simulink model "TRAMI_STEP_AT_vehicle_ver01_Jmaab_R2018b_Intg"  (R2018b)
settings: Solver=ode8  StartTime=0  StopTime=end_time  FixedStep=sampling_time  RelTol=1e-3
PreLoadFcn:
  | %init_setting;
values from neighbouring files (symbols this model uses):
  sampling_time = 0.0025    [METI_TRAMI_Thermal_ver01_Jmaab_PreLoad.m]
undefined symbols (not defined in the file or in its folder): ACC_D_Gain, ACC_I_Gain, ACC_P_Gain, ALT_CNT_ALT_OFF_RPM_HYS_rpm, ALT_CNT_ALT_ON_RPM_HYS_rpm, ALT_CNT_Alter_V_BASE_V, ALT_CNT_Alter_V_Kaisei_V, ALT_CNT_flag_disable_kaisei, ALT_CNT_V_Battely_Kudo_V, ALT_PNT_ALT_GDCurrent_A, ALT_PNT_ALT_GDVolt_V, ALT_PNT_Alter_limit_Current_V_table, ALT_PNT_Alter_limit_Current_V_table_x_rpm, ALT_PNT_Alter_trq_Nm_map, ALT_PNT_Alter_trq_Nm_map_x_rpm, ALT_PNT_Alter_trq_Nm_map_y_Current_A, ALT_PNT_Alter_trq_Nm_map_z_Volt_tgt_V, ALT_PNT_eta_pulley_alt, ALT_PNT_Gain_Alt_v_del, ALT_PNT_ratio_pulley_alt, ALT_PNT_Tau_Alternator_V_tgt_s, ALT_PNT_trq_alter_output_LL_Nm, BK_PNT_Pow_UL, BK_PNT_Tau_brake, Brk_LL, Brk_PGain, Brk_UL, BT_PNT_Lo_Capa_lo_batt_F, BT_PNT_Lo_ocv_SOC_lo_batt_OCV_V_table, BT_PNT_Lo_ocv_SOC_lo_batt_OCV_V_table_x_SOC, BT_PNT_Lo_R_lo_batt_ohm, BT_PNT_Lo_SOC_MAX_lo_batt, BT_PNT_Lo_SOC_MIN_lo_batt, BT_PNT_Lo_SOC_START_lo_batt, BT_PNT_Lo_V_start_ocv, Driver_Brake_Const1, Driver_Brake_Const3, Driver_Brake_Switch_Const2, Driver_Brk_sh, drivmode_ACC, drivmode_CONST, drivmode_GensokuKaisei, drivmode_GensokuRikko, drivmode_STOP, EL_PNT_R_bodyelec_lo_ohm, ENG_CNT_Accel_LL, ENG_CNT_Accel_UL, ENG_CNT_brak_idlestop, ENG_CNT_flag_idle_stop_exe, ENG_CNT_gain_p_per_isc, ENG_CNT_IdleSpeed_Const, ENG_CNT_omg_eng_fuelcut_rpm, ENG_CNT_per_isc_max, ENG_CNT_per_isc_min, ENG_CNT_per_throttle_fuelcut, ENG_CNT_per_throttle_isc_fb, ENG_CNT_Starter_timer_Const_s, ENG_CNT_Throttle_LL, ENG_CNT_Throttle_UL, ENG_CNT_V_car_idlestop_kmph ... (+29)
libraries: METI_Lib_vehicle_model x18, simulink x4, AZAPA_Lib_vehicle_model x1
(part 1 of 3)
settings Model: SimulationMode=accelerator  Creator=nishimura  LastModifiedBy=E00026
settings DataIOCC: LimitDataPoints=on  SaveFormat=Array  InspectSignalLogs=on
settings OptimizationCC: BlockReduction=off  BooleanDataType=off  LifeSpan=inf
settings DebuggingCC: SaveWithParameterizedLinksMsg=none  UnderspecifiedInitializationDetection=Classic  MergeDetectMultiDrivingBlocksExec=none  SignalResolutionControl=TryResolveAllWithWarning  ParameterPrecisionLossMsg=none  StrictBusMsg=ErrorOnBusTreatedAsVector  SFUnexpectedBacktrackingDiag=warning  SFNoUnconditionalDefaultTransitionDiag=warning  SFExecutionAtInitializationDiag=none
settings HardwareCC: ProdBitPerPointer=32  ProdBitPerSizeT=32  ProdBitPerPtrDiffT=32  ProdLargestAtomicFloat=None  ProdIntDivRoundTo=Undefined  ProdEndianess=Unspecified  ProdWordSize=32  ProdHWDeviceType=32-bit Generic  TargetUnknown=on
settings ModelReferenceCC: PropagateSignalLabelsOutOfModel=off
settings SFSimCC: SimUseLocalCustomCode=off
settings RTWCC: RTWUseLocalCustomCode=off
settings CodeAppCC: StateflowObjectComments=on
settings GRTTargetCC: TargetLangStandard=C89/C90 (ANSI)  GeneratePreprocessorConditionals=Disable all
settings ConfigComp: CovMetricSettings=dw  CovHtmlReporting=on  CovSaveCumulativeToWorkspaceVar=on  CovSaveSingleToWorkspaceVar=on  CovExternalEMLEnable=off  CovSFcnEnable=off

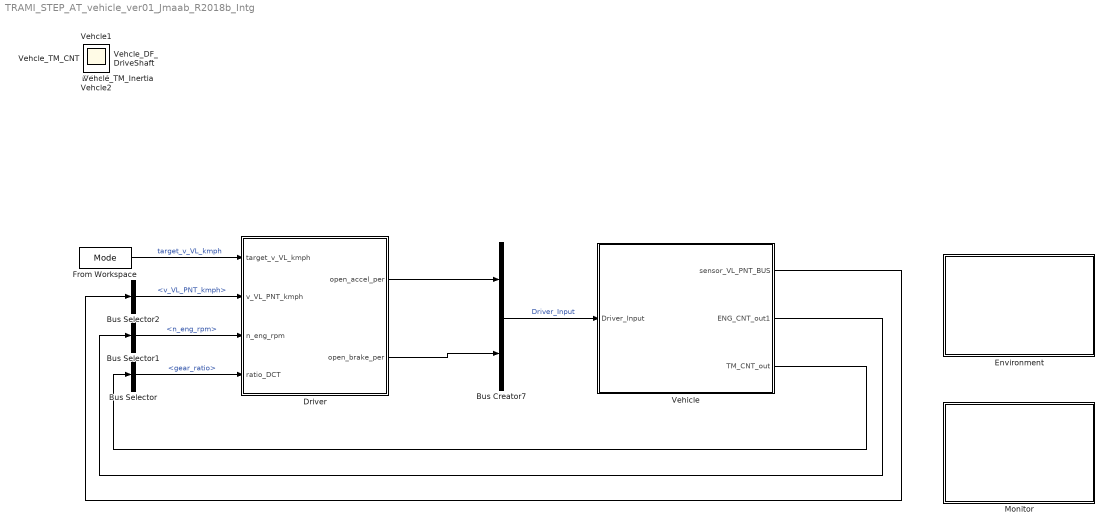
== system TRAMI_STEP_AT_vehicle_ver01_Jmaab_R2018b_Intg ==
  Bus Creator7 : BusCreator  Inputs=2
  Bus Selector : BusSelector  OutputSignals=gear_ratio
  Bus Selector1 : BusSelector  OutputSignals=n_eng_rpm
  Bus Selector2 : BusSelector  OutputSignals=v_VL_PNT_kmph
  Driver : Subsystem
      mask Display: image(imread('picture\driver.png'))
  Environment : Subsystem
      mask Display: image(imread('picture\environment.png'))
  From Workspace : FromWorkspace  VariableName=Mode  SampleTime=0  OutputAfterFinalValue=Holding final value
  Monitor : Subsystem
  Vehicle : Subsystem
      mask Display: image(imread('picture\electric_load.png'))
  Driver1 : Scope
  Vehcle1 : Scope
  Vehcle2 : Scope
  Vehcle_DF_DriveShaft : Scope
  Vehcle_TM_CNT : Scope
  Vehcle_TM_Inertia : Scope
  wires:
  From Workspace/1 -> Driver/1(target_v_VL_kmph)  "target_v_VL_kmph"
  Bus Creator7/1 -> Vehicle/1(Driver_Input)  "Driver_Input"
  Vehicle/1(sensor_VL_PNT_BUS) -> Bus Selector2/1
  Vehicle/3(TM_CNT_out) -> Bus Selector/1
  Vehicle/2(ENG_CNT_out1) -> Bus Selector1/1
  Driver/1(open_accel_per) -> Bus Creator7/1
  Driver/2(open_brake_per) -> Bus Creator7/2
  Bus Selector/1 -> Driver/4(ratio_DCT)  "<gear_ratio>"
  Bus Selector1/1 -> Driver/3(n_eng_rpm)  "<n_eng_rpm>"
  Bus Selector2/1 -> Driver/2(v_VL_PNT_kmph)  "<v_VL_PNT_kmph>"

== system TRAMI_STEP_AT_vehicle_ver01_Jmaab_R2018b_Intg/Driver ==
  note: ドライバモデルのへたくそ対応
  note: 全体としてパワーを算出しておいて、
      | さらにパワーと速度のF/Bを切り替えれるようにしておく
  target_v_VL_kmph : Inport
  v_VL_PNT_kmph : Inport  Port=2
  n_eng_rpm : Inport  Port=3
  ratio_DCT : Inport  Port=4
  Caliculate_Driving_State : Subsystem
  Caliculate_Opeining_Accel : Subsystem
  Caliculate_Opening_Brake : Subsystem
  Memory2 : Memory  InheritSampleTime=on
  Memory3 : Memory
  Memory4 : Memory
  open_accel_per : Outport
  open_brake_per : Outport  Port=2
  tag scope: tScope_accel=global, tScope_brake=global
  wires:
  target_v_VL_kmph/1 -> Caliculate_Opeining_Accel/2(target_v_VL_kmph), Caliculate_Opening_Brake/2(target_v_VL_kmph), Caliculate_Driving_State/2(target_v_VL_kmph)
  Memory3/1 -> Caliculate_Opeining_Accel/3(pre_n_eng_rpm)  "pre_n_eng_rpm"
  Memory4/1 -> Caliculate_Opeining_Accel/4(pre_ratio_DCT)
  n_eng_rpm/1 -> Memory3/1
  Memory2/1 -> Caliculate_Opening_Brake/1(v_VL_PNT_kmph), Caliculate_Opeining_Accel/1(v_VL_PNT_kmph)
  Caliculate_Opening_Brake/1(open_brake_per) -> open_brake_per/1, [tScope_brake], Caliculate_Driving_State/1(open_brake_per)
  v_VL_PNT_kmph/1 -> Memory2/1
  ratio_DCT/1 -> Memory4/1
  Caliculate_Opeining_Accel/1(open_accel_per) -> [tScope_accel], open_accel_per/1, Caliculate_Opening_Brake/3(open_accel_per)

== system TRAMI_STEP_AT_vehicle_ver01_Jmaab_R2018b_Intg/Environment ==
  note: 登坂。風、温度、湿度・・・
  Clock : Clock
  To Workspace : ToWorkspace  VariableName=simtime  SampleTime=-1
      settings: Decimation=num_tws_mabiki
  wires:
  Clock/1 -> To Workspace/1

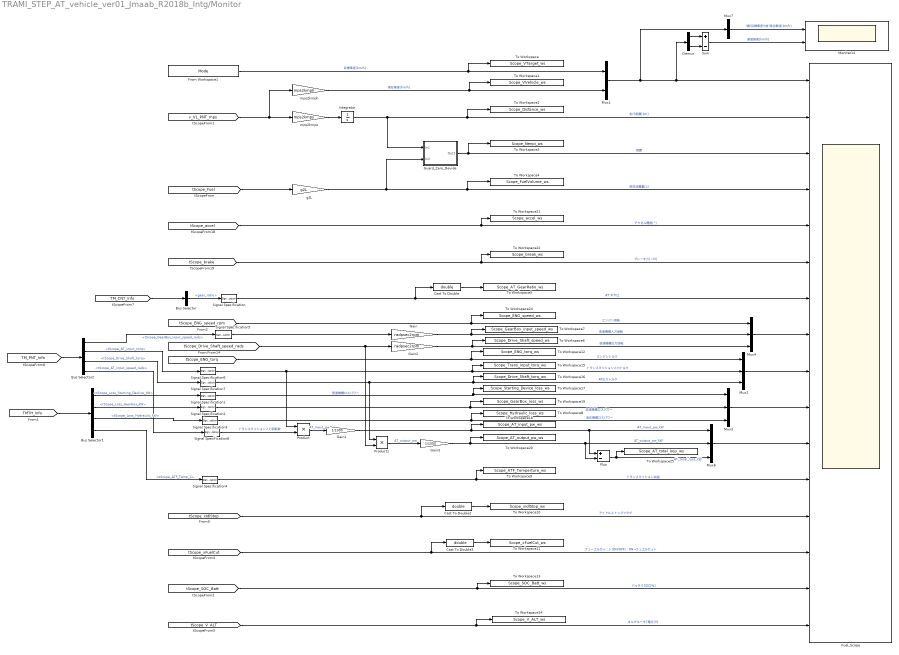
== system TRAMI_STEP_AT_vehicle_ver01_Jmaab_R2018b_Intg/Monitor ==
  Bus Selector : BusSelector  OutputSignals=gear_ratio
  Bus Selector1 : BusSelector  OutputSignals=tScope_Loss_Starting_Deviice_kW,tScope_Loss_Gearbox_kW,tScope_Loss_Hydraulic_kW,tScope_ATF_Temp_C
  Bus Selector2 : BusSelector  OutputSignals=tScope_GearBox_input_speed_rads,tScope_AT_input_torq,tScope_Drive_Shaft_torq,tScope_AT_input_speed_rads
  Cast To Double : DataTypeConversion  OutDataTypeStr=double
  Cast To Double2 : DataTypeConversion  OutDataTypeStr=double
  Cast To Double3 : DataTypeConversion  OutDataTypeStr=double
  Demux : Demux  Outputs=2
  From Workspace1 : FromWorkspace  VariableName=Mode  SampleTime=0  OutputAfterFinalValue=Holding final value
  Fuel_Scope : Scope  NumInputPorts=16
  Gain : Gain  Tag=単位変換  Gain=radpsec2rpm
  Gain1 : Gain  Gain=1/1000
  Gain2 : Gain  Tag=単位変換  Gain=radpsec2rpm
  Gain3 : Gain  Gain=1/1000
  Guard_Zero_Devide : Subsystem
  Integrator : Integrator
  Moniter14 : Scope  NumInputPorts=2
  Mux1 : Mux  Inputs=2
  Mux{2..4,6} (4 alike) : Mux  Inputs=3
  Mux7 : Mux  Inputs=1
  Plus : Sum  Inputs=+-
  Product : Product
  Product1 : Product
  Signal Specification{,1..8} (9 alike) : SignalSpecification
  Sum : Sum  Inputs=+-
  To Workspace : ToWorkspace  VariableName=Scope_VTarget_ws  SampleTime=-1
      settings: Decimation=num_tws_mabiki
  To Workspace1 : ToWorkspace  VariableName=Scope_VVehicle_ws  SampleTime=-1
      settings: Decimation=num_tws_mabiki
  To Workspace10 : ToWorkspace  VariableName=Scope_xIdlStop_ws  SampleTime=-1
      settings: Decimation=num_tws_mabiki
  To Workspace11 : ToWorkspace  VariableName=Scope_xFuelCut_ws  SampleTime=-1
      settings: Decimation=num_tws_mabiki
  To Workspace12 : ToWorkspace  VariableName=Scope_ENG_torq_ws  SampleTime=-1
      settings: Decimation=num_tws_mabiki
  To Workspace13 : ToWorkspace  VariableName=Scope_SOC_Batt_ws  SampleTime=-1
      settings: Decimation=num_tws_mabiki
  To Workspace14 : ToWorkspace  VariableName=Scope_V_ALT_ws  SampleTime=-1
      settings: Decimation=num_tws_mabiki
  To Workspace15 : ToWorkspace  VariableName=Scope_Trans_input_torq_ws  SampleTime=-1
      settings: Decimation=num_tws_mabiki
  To Workspace16 : ToWorkspace  VariableName=Scope_Drive_Shaft_torq_ws  SampleTime=-1
      settings: Decimation=num_tws_mabiki
  To Workspace17 : ToWorkspace  VariableName=Scope_Starting_Device_loss_ws  SampleTime=-1
      settings: Decimation=num_tws_mabiki
  To Workspace18 : ToWorkspace  VariableName=Scope_AT_input_pw_ws  SampleTime=-1
      settings: Decimation=num_tws_mabiki
  To Workspace19 : ToWorkspace  VariableName=Scope_GearBox_loss_ws  SampleTime=-1
      settings: Decimation=num_tws_mabiki
  To Workspace2 : ToWorkspace  VariableName=Scope_Distance_ws  SampleTime=-1
      settings: Decimation=num_tws_mabiki
  To Workspace20 : ToWorkspace  VariableName=Scope_AT_output_pw_ws  SampleTime=-1
      settings: Decimation=num_tws_mabiki
  To Workspace21 : ToWorkspace  VariableName=Scope_accel_ws  SampleTime=-1
      settings: Decimation=num_tws_mabiki
  To Workspace22 : ToWorkspace  VariableName=Scope_break_ws  SampleTime=-1
      settings: Decimation=num_tws_mabiki
  To Workspace24 : ToWorkspace  VariableName=Scope_ENG_speed_ws  SampleTime=-1
      settings: Decimation=num_tws_mabiki
  To Workspace25 : ToWorkspace  VariableName=Scope_AT_total_loss_ws  SampleTime=-1
      settings: Decimation=num_tws_mabiki
  To Workspace3 : ToWorkspace  VariableName=Scope_Nenpi_ws  SampleTime=-1
      settings: Decimation=num_tws_mabiki
  To Workspace4 : ToWorkspace  VariableName=Scope_FuelVolume_ws  SampleTime=-1
      settings: Decimation=num_tws_mabiki
  To Workspace5 : ToWorkspace  VariableName=Scope_AT_GearRatio_ws  SampleTime=-1
      settings: Decimation=num_tws_mabiki
  To Workspace6 : ToWorkspace  VariableName=Scope_Drive_Shaft_speed_ws  SampleTime=-1
      settings: Decimation=num_tws_mabiki
  To Workspace7 : ToWorkspace  VariableName=Scope_GearBox_input_speed_ws  SampleTime=-1
      settings: Decimation=num_tws_mabiki
  To Workspace8 : ToWorkspace  VariableName=Scope_Hydraulic_loss_ws  SampleTime=-1
      settings: Decimation=num_tws_mabiki
  To Workspace9 : ToWorkspace  VariableName=Scope_ATF_Temperture_ws  SampleTime=-1
      settings: Decimation=num_tws_mabiki
  g2L : Gain  Gain=g2L
  mps2kmph : Gain  Gain=mps2kmph
  mps2kmps : Gain  Gain=mps2kmps
  wires:
  [tScope_xFuelCut] -> Fuel_Scope/14, Cast To Double3/1  "フューエルカット[ON/OFF] : ON→フュエルカット"
  [v_VL_PNT_mps] -> mps2kmph/1, mps2kmps/1
  mps2kmps/1 -> Integrator/1
  [tScope_Fuel] -> g2L/1
  Integrator/1 -> Guard_Zero_Devide/1(In1), Fuel_Scope/2, To Workspace2/1  "走行距離[km]"
  g2L/1 -> Fuel_Scope/4, To Workspace4/1, Guard_Zero_Devide/2(In2)  "燃料消費量[L]"
  Signal Specification4/1 -> Fuel_Scope/12, To Workspace9/1  "トランスミッション油温"
  From Workspace1/1 -> To Workspace/1, Mux1/1  "目標車速[km/h]"
  mps2kmph/1 -> To Workspace1/1, Mux1/2  "現在車速[km/h]"
  Mux1/1 -> Mux7/1, Fuel_Scope/1, Demux/1
  Signal Specification2/1 -> To Workspace19/1, Mux3/2  "変速機構ロスパワー"
  Signal Specification7/1 -> Product1/1, To Workspace16/1, Mux2/3  "AT出力トルク"
  Mux3/1 -> Fuel_Scope/10
  [tScope_accel] -> Fuel_Scope/5, To Workspace21/1  "アクセル開度[°]"
  [tScope_brake] -> Fuel_Scope/6, To Workspace22/1  "ブレーキ力[１N]"
  [tScope_ENG_speed_rpm] -> To Workspace24/1, Mux4/1  "エンジン回転"
  Demux/1 -> Sum/1
  Demux/2 -> Sum/2
  Sum/1 -> Moniter14/2  "速度誤差[km/h]"
  [tScope_V_ALT] -> Fuel_Scope/16, To Workspace14/1  "オルタネータ7電圧[V]"
  [tScope_SOC_Batt] -> Fuel_Scope/15, To Workspace13/1  "バッテリSOC[%]"
  Guard_Zero_Devide/1(Out1) -> Fuel_Scope/3, To Workspace3/1  "燃費"
  Gain/1 -> Mux4/2, To Workspace7/1  "変速機構入力回転"
  [tScope_ENG_torq] -> To Workspace12/1, Mux2/1  "エンジントルク"
  Signal Specification6/1 -> Mux2/2, To Workspace15/1, Product/1  "トランスミッション入力トルク"
  Signal Specification1/1 -> To Workspace17/1, Mux3/1  "発進機構ロスパワー"
  Signal Specification3/1 -> To Workspace8/1, Mux3/3  "油圧機構ロスパワー"
  Mux2/1 -> Fuel_Scope/9
  [tScope_xIdlStop] -> Fuel_Scope/13, Cast To Double2/1  "アイドルストップフラグ"
  Mux4/1 -> Fuel_Scope/8
  Cast To Double3/1 -> To Workspace11/1
  Cast To Double2/1 -> To Workspace10/1
  Signal Specification5/1 -> Gain/1
  Gain2/1 -> To Workspace6/1, Mux4/3  "変速機構出力回転"
  [tScope_Drive_Shaft_speed_rads] -> Product1/2, Gain2/1
  Mux6/1 -> Fuel_Scope/11
  Gain1/1 -> To Workspace18/1, Mux6/1, Plus/1  "AT_Input_pw_kW"
  Signal Specification8/1 -> Product/2  "トランスミッション入力回転数"
  Product1/1 -> Gain3/1  "AT_output_pw"
  Plus/1 -> To Workspace25/1, Mux6/3  "AT_total_loss_kW"
  Product/1 -> Gain1/1  "AT_Input_pw"
  Gain3/1 -> To Workspace20/1, Plus/2, Mux6/2  "AT_output_pw_kW"
  Cast To Double/1 -> To Workspace5/1
  Signal Specification/1 -> Cast To Double/1, Fuel_Scope/7  "AT ギヤ比"
  Mux7/1 -> Moniter14/1  "(黄)目標車速/(桃)現在車速[km/h]"
  [TM_CNT_Info] -> Bus Selector/1
  Bus Selector/1 -> Signal Specification/1  "<gear_ratio>"
  [TMTH_Info] -> Bus Selector1/1
  Bus Selector1/1 -> Signal Specification1/1  "<tScope_Loss_Starting_Deviice_kW>"
  Bus Selector1/2 -> Signal Specification2/1  "<tScope_Loss_Gearbox_kW>"
  Bus Selector1/3 -> Signal Specification3/1  "<tScope_Loss_Hydraulic_kW>"
  Bus Selector1/4 -> Signal Specification4/1  "<tScope_ATF_Temp_C>"
  [TM_PNT_Info] -> Bus Selector2/1
  Bus Selector2/1 -> Signal Specification5/1  "<tScope_GearBox_input_speed_rads>"
  Bus Selector2/2 -> Signal Specification6/1  "<tScope_AT_input_torq>"
  Bus Selector2/3 -> Signal Specification7/1  "<tScope_Drive_Shaft_torq>"
  Bus Selector2/4 -> Signal Specification8/1  "<tScope_AT_input_speed_rads>"

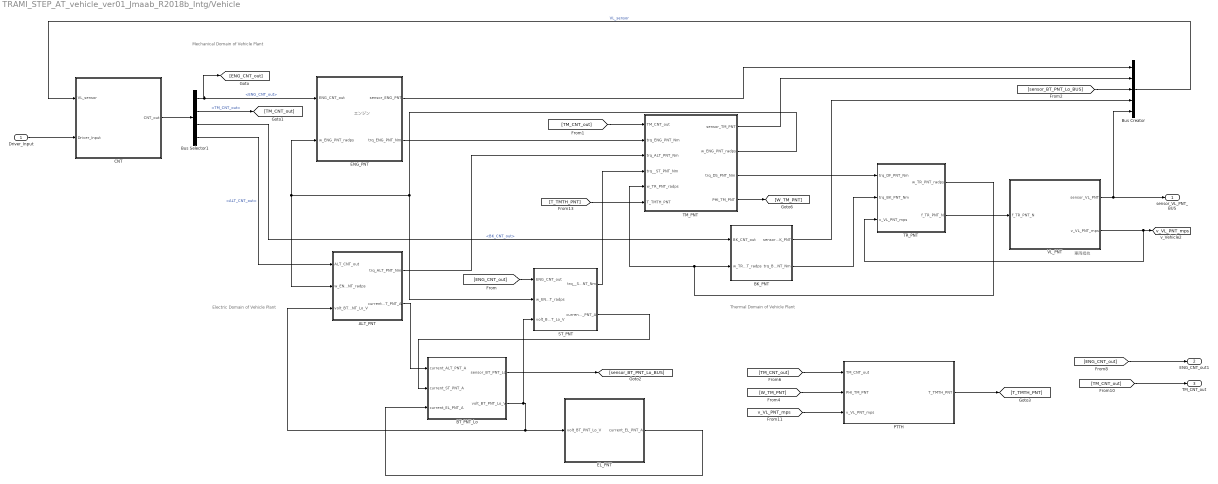
== system TRAMI_STEP_AT_vehicle_ver01_Jmaab_R2018b_Intg/Vehicle ==
  note: エンジン
  note: 車両抵抗
  note: Mechanical Domain of Vehicle Plant
  note: Electric Domain
      |  of Vehicle Plant
  note: Thermal Domain of Vehicle Plant
  Driver_Input : Inport
  ALT_PNT : Subsystem
      mask Display: image(imread('picture\image\alternator02.jpg'))
  BK_PNT : Subsystem
      mask Display: image(imread('picture\brake02.png'))
  BT_PNT_Lo : Subsystem
      mask Display: image(imread('picture\battery.png'))
  Bus Creator : BusCreator  Inputs=5
  Bus Selector1 : BusSelector  OutputSignals=ENG_CNT_out,TM_CNT_out,BK_CNT_out,ALT_CNT_out
  CNT : Subsystem
      mask Display: image(imread('picture\ECU.png'))
  EL_PNT : Subsystem
      mask Display: image(imread('picture\electric_load.png'))
  ENG_PNT : Subsystem
      mask Display: image(imread('picture\image\engine03.jpg'))
  PTTH : Subsystem
  ST_PNT : Subsystem
      mask Display: image(imread('picture\image\starter02.jpg'))
  TM_PNT : Subsystem
  TR_PNT : Subsystem
      mask Display: image(imread('picture\tyre01.png'))
  VL_PNT : Subsystem
      mask Display: image(imread('picture\vehicle_resistance.png'))
  sensor_VL_PNT_BUS : Outport
  ENG_CNT_out1 : Outport  Port=2
  TM_CNT_out : Outport  Port=3
  tag scope: v_VL_PNT_mps=global
  wires:
  ENG_PNT/1(sensor_ENG_PNT) -> Bus Creator/1
  ALT_PNT/1(trq_ALT_PNT_Nm) -> TM_PNT/3(trq_ALT_PNT_Nm)
  EL_PNT/1(current_EL_PNT_A) -> BT_PNT_Lo/3(current_EL_PNT_A)
  ALT_PNT/2(current_ALT_PNT_A) -> BT_PNT_Lo/1(current_ALT_PNT_A)
  ST_PNT/2(current_ST_PNT_A) -> BT_PNT_Lo/2(current_ST_PNT_A)
  BT_PNT_Lo/2(volt_BT_PNT_Lo_V) -> ST_PNT/3(volt_BT_PNT_Lo_V), ALT_PNT/3(volt_BT_PNT_Lo_V), EL_PNT/1(volt_BT_PNT_Lo_V)
  TM_PNT/1(sensor_TM_PNT) -> Bus Creator/2
  ENG_PNT/2(trq_ENG_PNT_Nm) -> TM_PNT/2(trq_ENG_PNT_Nm)
  TM_PNT/2(w_ENG_PNT_radps) -> ALT_PNT/2(w_ENG_PNT_radps), ENG_PNT/2(w_ENG_PNT_radps), ST_PNT/2(w_ENG_PNT_radps)
  ST_PNT/1(trq__ST_PNT_Nm) -> TM_PNT/4(trq__ST_PNT_Nm)
  VL_PNT/1(sensor_VL_PNT) -> sensor_VL_PNT_BUS/1, Bus Creator/5
  TM_PNT/3(trq_DS_PNT_Nm) -> TR_PNT/1(trq_DF_PNT_Nm)
  BK_PNT/2(trq_BK_PNT_Nm) -> TR_PNT/2(trq_BK_PNT_Nm)
  TR_PNT/2(f_TR_PNT_N) -> VL_PNT/1(f_TR_PNT_N)
  TR_PNT/1(w_TR_PNT_radps) -> TM_PNT/5(w_TR_PNT_radps), BK_PNT/2(w_TR_PNT_radps)
  VL_PNT/2(v_VL_PNT_mps) -> TR_PNT/3(v_VL_PNT_mps), [v_VL_PNT_mps]
  [TM_CNT_out] -> TM_CNT_out/1
  Bus Selector1/1 -> [ENG_CNT_out], ENG_PNT/1(ENG_CNT_out)  "<ENG_CNT_out>"
  Bus Selector1/4 -> ALT_PNT/1(ALT_CNT_out)  "<ALT_CNT_out>"
  Bus Selector1/3 -> BK_PNT/1(BK_CNT_out)  "<BK_CNT_out>"
  Bus Creator/1 -> CNT/1(VL_sensor)  "VL_sensor"
  CNT/1(CNT_out) -> Bus Selector1/1
  [ENG_CNT_out] -> ST_PNT/1(ENG_CNT_out)
  Bus Selector1/2 -> [TM_CNT_out]  "<TM_CNT_out>"
  [TM_CNT_out] -> TM_PNT/1(TM_CNT_out)
  BT_PNT_Lo/1(sensor_BT_PNT_Lo) -> [sensor_BT_PNT_Lo_BUS]
  [sensor_BT_PNT_Lo_BUS] -> Bus Creator/3
  Driver_Input/1 -> CNT/2(Driver_Input)
  [ENG_CNT_out] -> ENG_CNT_out1/1
  PTTH/1(T_TMTH_PNT) -> [T_TMTH_PNT]
  [TM_CNT_out] -> PTTH/1(TM_CNT_out)
  [W_TM_PNT] -> PTTH/2(PHI_TM_PNT)
  [v_VL_PNT_mps] -> PTTH/3(v_VL_PNT_mps)
  TM_PNT/4(PHI_TM_PNT) -> [W_TM_PNT]
  [T_TMTH_PNT] -> TM_PNT/6(T_TMTH_PNT)
  BK_PNT/1(sensor_BK_PNT) -> Bus Creator/4

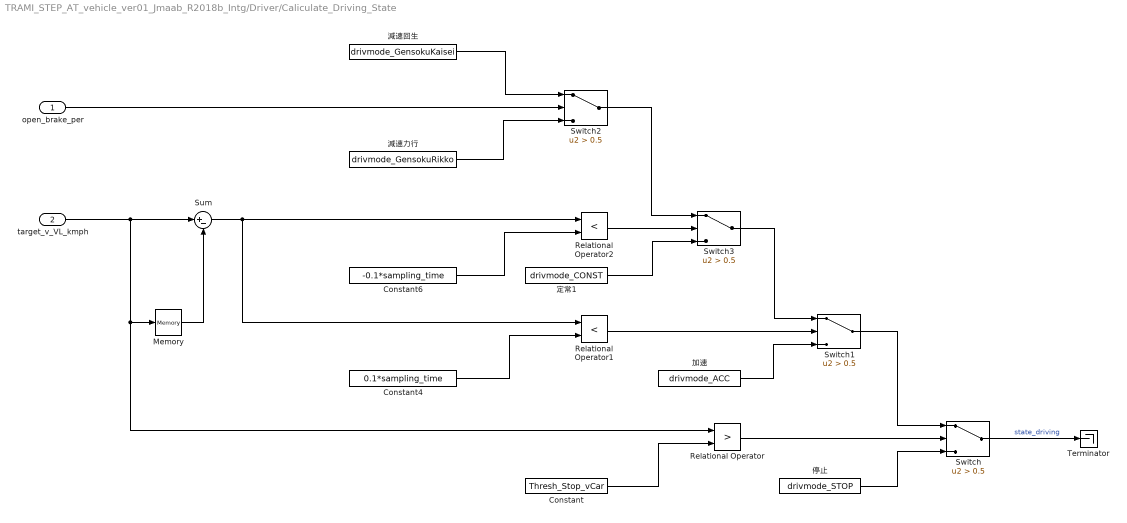
== system TRAMI_STEP_AT_vehicle_ver01_Jmaab_R2018b_Intg/Driver/Caliculate_Driving_State ==
  open_brake_per : Inport
  target_v_VL_kmph : Inport  Port=2
  Constant : Constant  Value=Thresh_Stop_vCar
  Constant4 : Constant  Value=0.1*sampling_time
  Constant6 : Constant  Value=-0.1*sampling_time
  Memory : Memory
  Relational Operator : RelationalOperator  Operator=>  OutDataTypeStr=boolean  RndMeth=Nearest
  Relational Operator1 : RelationalOperator  Operator=<  OutDataTypeStr=boolean  RndMeth=Nearest
  Relational Operator2 : RelationalOperator  Operator=<  OutDataTypeStr=boolean  RndMeth=Nearest
  Sum : Sum  Inputs=|+-
  Switch{,1..3} (4 alike) : Switch  Criteria=u2 > Threshold  Threshold=0.5
  Terminator : Terminator
  停止 : Constant  Value=drivmode_STOP
  加速 : Constant  Value=drivmode_ACC
  定常1 : Constant  Value=drivmode_CONST
  減速力行 : Constant  Value=drivmode_GensokuRikko
  減速回生 : Constant  Value=drivmode_GensokuKaisei
  wires:
  Switch/1 -> Terminator/1  "state_driving"
  target_v_VL_kmph/1 -> Relational Operator/1, Memory/1, Sum/1
  Relational Operator1/1 -> Switch1/2
  Constant4/1 -> Relational Operator1/2
  Relational Operator/1 -> Switch/2
  Constant/1 -> Relational Operator/2
  停止/1 -> Switch/3
  Sum/1 -> Relational Operator1/1, Relational Operator2/1
  減速回生/1 -> Switch2/1
  Switch3/1 -> Switch1/1
  Constant6/1 -> Relational Operator2/2
  Memory/1 -> Sum/2
  open_brake_per/1 -> Switch2/2
  減速力行/1 -> Switch2/3
  Relational Operator2/1 -> Switch3/2
  Switch2/1 -> Switch3/1
  定常1/1 -> Switch3/3
  加速/1 -> Switch1/3
  Switch1/1 -> Switch/1

== system TRAMI_STEP_AT_vehicle_ver01_Jmaab_R2018b_Intg/Driver/Caliculate_Opeining_Accel ==
  v_VL_PNT_kmph : Inport
  target_v_VL_kmph : Inport  Port=2
  pre_n_eng_rpm : Inport  Port=3
  pre_ratio_DCT : Inport  Port=4
  FB : Subsystem  mask{P_Gain=ACC_P_Gain, D_Gain=ACC_D_Gain, I_Gain=ACC_I_Gain}
      mask prompts: P_Gain "Pゲイン値"; D_Gain "Dゲイン値"; I_Gain "Iゲイン値"
  FF : Subsystem
  Guard_0_100 : Saturate  UpperLimit=ENG_CNT_Throttle_UL  LowerLimit=ENG_CNT_Throttle_LL
  Sum1 : Sum  Inputs=|-+
  Sum3 : Sum  Inputs=++|
  open_accel_per : Outport
  wires:
  Sum1/1 -> FB/1(delta_v_VL_kmph)
  v_VL_PNT_kmph/1 -> FF/1(v_VL_PNT_kmph), Sum1/1
  target_v_VL_kmph/1 -> FF/2(target_v_VL_kmph), Sum1/2
  Sum3/1 -> Guard_0_100/1
  pre_n_eng_rpm/1 -> FF/3(pre_n_eng_rpm)
  pre_ratio_DCT/1 -> FF/4(pre_ratio_DCT)
  FB/1(FB_open_accel_per) -> Sum3/1
  FF/1(FF_open_accel_per) -> Sum3/2
  Guard_0_100/1 -> open_accel_per/1  "open_accel_per"

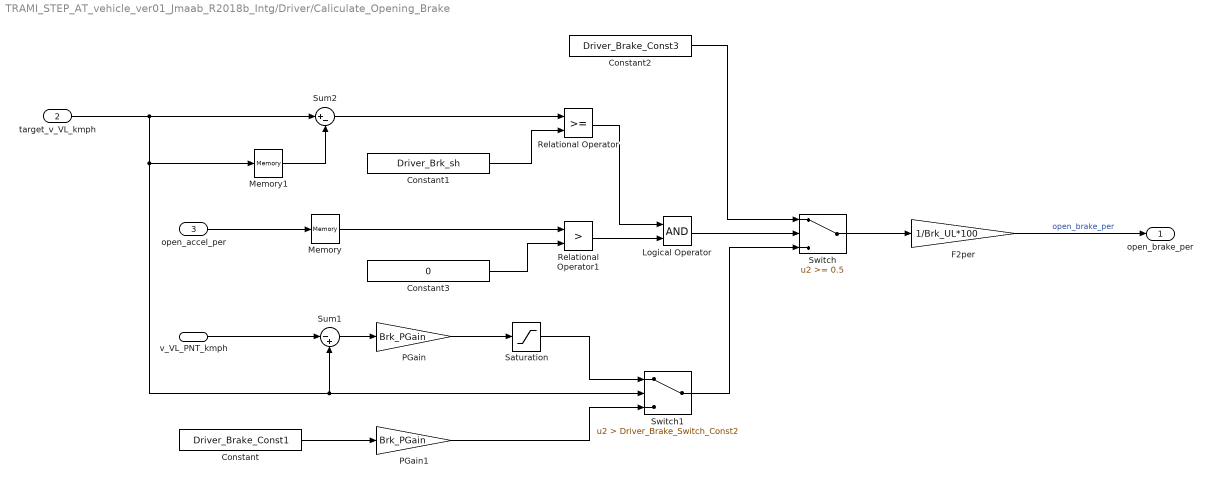
== system TRAMI_STEP_AT_vehicle_ver01_Jmaab_R2018b_Intg/Driver/Caliculate_Opening_Brake ==
  v_VL_PNT_kmph : Inport
  target_v_VL_kmph : Inport  Port=2
  open_accel_per : Inport  Port=3
  Constant : Constant  Value=Driver_Brake_Const1
  Constant1 : Constant  Value=Driver_Brk_sh
  Constant2 : Constant  Value=Driver_Brake_Const3
  Constant3 : Constant  Value=0
  F2per : Gain  Gain=1/Brk_UL*100
  Logical Operator : Logic  AllPortsSameDT=off  OutDataTypeStr=boolean
  Memory : Memory
  Memory1 : Memory
  PGain : Gain  Gain=Brk_PGain
  PGain1 : Gain  Gain=Brk_PGain
  Relational Operator : RelationalOperator  OutDataTypeStr=boolean  RndMeth=Nearest
  Relational Operator1 : RelationalOperator  Operator=>  OutDataTypeStr=boolean  RndMeth=Nearest
  Saturation : Saturate  UpperLimit=Brk_UL  LowerLimit=Brk_LL
  Sum1 : Sum  Inputs=|-+
  Sum2 : Sum  Inputs=|+-
  Switch : Switch  Threshold=0.5
  Switch1 : Switch  Criteria=u2 > Threshold  Threshold=Driver_Brake_Switch_Const2
  open_brake_per : Outport
  wires:
  target_v_VL_kmph/1 -> Switch1/2, Sum1/2, Memory1/1, Sum2/1
  Sum1/1 -> PGain/1
  PGain/1 -> Saturation/1
  Constant/1 -> PGain1/1
  PGain1/1 -> Switch1/3
  open_accel_per/1 -> Memory/1
  Memory/1 -> Relational Operator1/1
  Memory1/1 -> Sum2/2
  Switch/1 -> F2per/1
  Sum2/1 -> Relational Operator/1
  Saturation/1 -> Switch1/1
  Switch1/1 -> Switch/3
  Constant2/1 -> Switch/1
  v_VL_PNT_kmph/1 -> Sum1/1
  Constant1/1 -> Relational Operator/2
  Constant3/1 -> Relational Operator1/2
  Relational Operator1/1 -> Logical Operator/2
  Relational Operator/1 -> Logical Operator/1
  Logical Operator/1 -> Switch/2
  F2per/1 -> open_brake_per/1  "open_brake_per"

== system TRAMI_STEP_AT_vehicle_ver01_Jmaab_R2018b_Intg/Monitor/Guard_Zero_Devide ==
  note: 0割防止暫定処置
  In1 : Inport
  In2 : Inport  Port=2
  Constant1 : Constant  Value=fuel_0guard
  Constant2 : Constant  Value=fuelcomsnp_0
  Divide : Product  Inputs=*/
  MinMax : MinMax  Function=max  Inputs=2
  Relational Operator : RelationalOperator  OutDataTypeStr=boolean  RndMeth=Nearest
  Switch1 : Switch  Criteria=u2 > Threshold  Threshold=0.5
  Out1 : Outport
  wires:
  In2/1 -> MinMax/1, Relational Operator/1
  In1/1 -> Divide/1
  Switch1/1 -> Out1/1  "燃費[km/l]"
  Divide/1 -> Switch1/1  "燃費[km/l]"
  Constant2/1 -> Switch1/3
  Relational Operator/1 -> Switch1/2
  MinMax/1 -> Divide/2
  Constant1/1 -> MinMax/2, Relational Operator/2

== system TRAMI_STEP_AT_vehicle_ver01_Jmaab_R2018b_Intg/Vehicle/ALT_PNT ==
  note: 発電する為のトルクが負
  note: スルー量が出力の場合、発電する方向が正
  ALT_CNT_out : Inport
  w_ENG_PNT_radps : Inport  Port=2
  volt_BT_PNT_Lo_V : Inport  Port=3
  Bus Selector8 : BusSelector  OutputSignals=target_volt_ALT_V
  Gain : Gain  Gain=-1
  Memory1 : Memory
  P_cal : METI_Lib_vehicle_model/P_cal  Type_energy=回転運動  Type_output_energy=出力  Power_name=Po_  t_Workspace_Name=ALT_PNT_MECK  P_VariableName=Po_ALT_PNT_MECK  Across_VariableName=w_ALT_PNT_MECK  Throgh_VariableName=tq_ALT_PNT_MECK
  P_cal1 : METI_Lib_vehicle_model/P_cal  Type_energy=電気  Type_output_energy=出力  Power_name=Po_  t_Workspace_Name=ALT_PNT_ELEC  P_VariableName=Po_ALT_PNT_ELEC  Across_VariableName=V_ALT_PNT_ELEC  Throgh_VariableName=I_ALT_PNT_ELEC
  Subsystem : Subsystem
  Terminator : Terminator
  Terminator1 : Terminator
  pulley_slave : Subsystem
  trq_ALT_PNT_Nm : Outport
  current_ALT_PNT_A : Outport  Port=2
  tag scope: tScope_V_ALT=global
  wires:
  Memory1/1 -> Subsystem/2(w_ROT_slavepulley12)
  Subsystem/1(current_ALT_PNT_A) -> P_cal1/2, current_ALT_PNT_A/1
  Gain/1 -> trq_ALT_PNT_Nm/1  "trq_ALT_PNT_Nm"
  pulley_slave/1(trq_slavepulley11) -> Gain/1
  w_ENG_PNT_radps/1 -> pulley_slave/1(w_ENG_PNT_radps)
  Subsystem/2(trq_trqsource) -> P_cal/2, pulley_slave/2(trq_slavepulley12)
  volt_BT_PNT_Lo_V/1 -> [tScope_V_ALT], P_cal1/1, Subsystem/3(volt_BT_PNT_Lo_V)
  P_cal1/1 -> Terminator1/1
  P_cal/1 -> Terminator/1
  pulley_slave/2(w_slavepulley12) -> P_cal/1, Memory1/1
  ALT_CNT_out/1 -> Bus Selector8/1
  Bus Selector8/1 -> Subsystem/1(target_volt_ALT_V)  "<target_volt_ALT_V>"

== system TRAMI_STEP_AT_vehicle_ver01_Jmaab_R2018b_Intg/Vehicle/BK_PNT ==
  note: 制動力
  BK_CNT_out : Inport
  w_TR_PNT_radps : Inport  Port=2
  Bus Creator : BusCreator  Inputs=1
  Bus Selector : BusSelector  OutputSignals=open_brake_per
  Constant2 : Constant  Value=tire_r
  Gain : Gain  Gain=-1
  Product6 : Product  RndMeth=Zero
  Q_cal3 : METI_Lib_vehicle_model/P_cal  Type_energy=回転運動  Type_output_energy=損失  Power_name=Pl_  t_Workspace_Name=BK_PNT_MECK_LOSS  P_VariableName=Pl_BK_PNT_MECK_LOSS  Across_VariableName=w_BK_PNT_MECK_LOSS  Throgh_VariableName=tq_BK_PNT_MECK_LOSS
  Terminator1 : Terminator
  Transfer Fcn : TransferFcn  Denominator=[BK_PNT_Tau_brake 1]
  per2F : Gain  Gain=BK_PNT_Pow_UL/100
  sensor_BK_PNT : Outport
  trq_BK_PNT_Nm : Outport  Port=2
  wires:
  Q_cal3/1 -> Terminator1/1
  Transfer Fcn/1 -> Product6/2
  Constant2/1 -> Product6/1
  Product6/1 -> Gain/1, Q_cal3/2
  w_TR_PNT_radps/1 -> Q_cal3/1
  BK_CNT_out/1 -> Bus Selector/1
  Gain/1 -> Bus Creator/1, trq_BK_PNT_Nm/1  "trq_BK_PNT_Nm"
  per2F/1 -> Transfer Fcn/1
  Bus Selector/1 -> per2F/1  "<open_brake_per>"
  Bus Creator/1 -> sensor_BK_PNT/1  "sensor_BK_PNT"

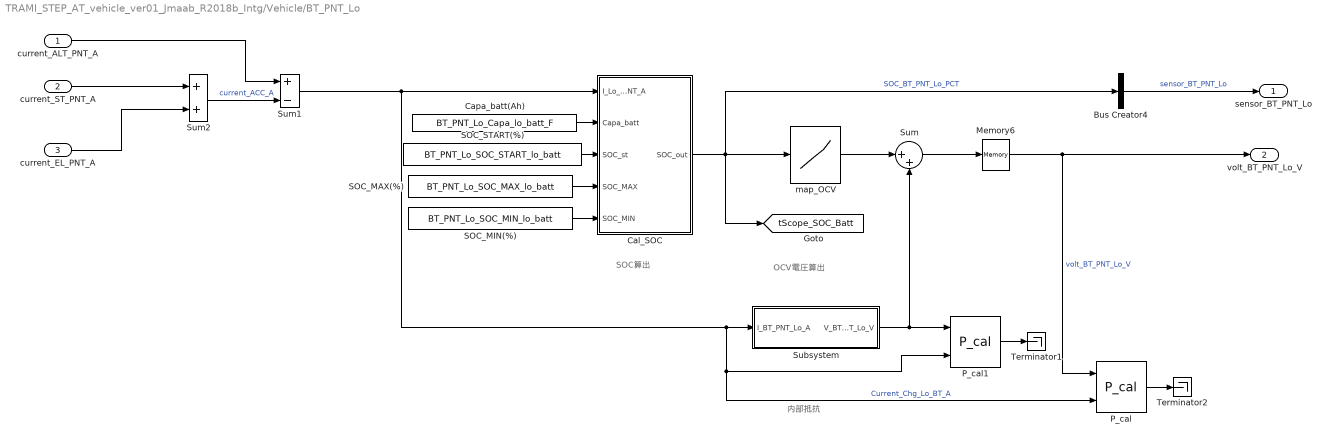
== system TRAMI_STEP_AT_vehicle_ver01_Jmaab_R2018b_Intg/Vehicle/BT_PNT_Lo ==
  note: SOC算出
  note: 内部抵抗
  note: OCV電圧算出
  current_ALT_PNT_A : Inport
  current_ST_PNT_A : Inport  Port=2
  current_EL_PNT_A : Inport  Port=3
  Bus Creator4 : BusCreator  Inputs=1
  Cal_SOC : Subsystem
  Capa_batt(Ah) : Constant  Value=BT_PNT_Lo_Capa_lo_batt_F
  Memory6 : Memory  InitialCondition=BT_PNT_Lo_V_start_ocv  InheritSampleTime=on
  P_cal : METI_Lib_vehicle_model/P_cal  Type_energy=電気  Type_output_energy=出力  Power_name=Po_  t_Workspace_Name=BT_PNT_Lo_ELEC  P_VariableName=Po_BT_PNT_Lo_ELEC  Across_VariableName=V_BT_PNT_Lo_ELEC  Throgh_VariableName=I_BT_PNT_Lo_ELEC
  P_cal1 : METI_Lib_vehicle_model/P_cal  Type_energy=電気  Type_output_energy=損失  Power_name=Pl_  t_Workspace_Name=BT_PNT_Lo_ELEC_LOSS  P_VariableName=Pl_BT_PNT_Lo_ELEC_LOSS  Across_VariableName=V_BT_PNT_Lo_ELEC_LOSS  Throgh_VariableName=I_BT_PNT_Lo_ELEC_LOSS
  SOC_MAX(%) : Constant  Value=BT_PNT_Lo_SOC_MAX_lo_batt
  SOC_MIN(%) : Constant  Value=BT_PNT_Lo_SOC_MIN_lo_batt
  SOC_START(%) : Constant  Value=BT_PNT_Lo_SOC_START_lo_batt
  Subsystem : Subsystem
  Sum : Sum  Inputs=|++
  Sum1 : Sum  Inputs=+-
  Sum2 : Sum
  Terminator1 : Terminator
  Terminator2 : Terminator
  map_OCV : Lookup  InputValues=BT_PNT_Lo_ocv_SOC_lo_batt_OCV_V_table_x_SOC  Table=BT_PNT_Lo_ocv_SOC_lo_batt_OCV_V_table  LookUpMeth=Interpolation-Use End Values
  sensor_BT_PNT_Lo : Outport
  volt_BT_PNT_Lo_V : Outport  Port=2
  tag scope: tScope_SOC_Batt=global
  wires:
  Sum/1 -> Memory6/1
  Capa_batt(Ah)/1 -> Cal_SOC/2(Capa_batt)
  SOC_START(%)/1 -> Cal_SOC/3(SOC_st)
  SOC_MAX(%)/1 -> Cal_SOC/4(SOC_MAX)
  SOC_MIN(%)/1 -> Cal_SOC/5(SOC_MIN)
  Memory6/1 -> volt_BT_PNT_Lo_V/1, P_cal/1  "volt_BT_PNT_Lo_V"
  map_OCV/1 -> Sum/1
  Subsystem/1(V_BT_PNT_Lo_V) -> P_cal1/1, Sum/2
  P_cal/1 -> Terminator2/1
  P_cal1/1 -> Terminator1/1
  Cal_SOC/1(SOC_out) -> Bus Creator4/1, map_OCV/1, [tScope_SOC_Batt]  "SOC_BT_PNT_Lo_PCT"
  Bus Creator4/1 -> sensor_BT_PNT_Lo/1  "sensor_BT_PNT_Lo"
  Sum1/1 -> P_cal/2, P_cal1/2, Subsystem/1(I_BT_PNT_Lo_A), Cal_SOC/1(I_Lo_BT_PNT_A)  "Current_Chg_Lo_BT_A"
  Sum2/1 -> Sum1/2  "current_ACC_A"
  current_ALT_PNT_A/1 -> Sum1/1
  current_ST_PNT_A/1 -> Sum2/1
  current_EL_PNT_A/1 -> Sum2/2

== system TRAMI_STEP_AT_vehicle_ver01_Jmaab_R2018b_Intg/Vehicle/CNT ==
  note: Control Model
  note: Gtoto From Tag Visibility for CAN
  VL_sensor : Inport
  Driver_Input : Inport  Port=2
  ALT_CNT : Subsystem
  BK_CNT : Subsystem
  Bus Creator1 : BusCreator  Inputs=4
  Bus Selector : BusSelector  OutputSignals=sensor_ENG_PNT,sensor_TM_PNT,sensor_BT_PNT_Lo,sensor_VL_PNT,sensor_BK_PNT
  CAN : Subsystem
  ENG_CNT : Subsystem
  Goto Tag Visibility : GotoTagVisibility  GotoTag=ENG_CNT_CAN_Tx
  Goto Tag Visibility1 : GotoTagVisibility  GotoTag=TM_CNT_CAN_Tx
  Goto Tag Visibility2 : GotoTagVisibility  GotoTag=ALT_CNT_CAN_Rx
  Goto Tag Visibility3 : GotoTagVisibility  GotoTag=ENG_CNT_CAN_Rx
  Goto Tag Visibility4 : GotoTagVisibility  GotoTag=TM_CNT_CAN_Rx
  Goto Tag Visibility5 : GotoTagVisibility  GotoTag=BK_CNT_CAN_Tx
  TM_CNT : Subsystem
  CNT_out : Outport
  wires:
  Bus Creator1/1 -> CNT_out/1  "CNT_out"
  Bus Selector/4 -> BK_CNT/2(sensor_VL_PNT)  "<sensor_VL_PNT>"
  VL_sensor/1 -> Bus Selector/1
  Bus Selector/3 -> ALT_CNT/1(sensor_BT_PNT_Lo_BUS)  "<sensor_BT_PNT_Lo>"
  Bus Selector/2 -> TM_CNT/1(sensor_TM_PNT_BUS)  "<sensor_TM_PNT>"
  Bus Selector/1 -> ENG_CNT/2(sensor_ENG_PNT)  "<sensor_ENG_PNT>"
  ALT_CNT/1(ALT_CNT_out) -> Bus Creator1/3
  ENG_CNT/1(ENG_CNT_out) -> Bus Creator1/1
  TM_CNT/1(TM_CNT_out) -> Bus Creator1/2
  Driver_Input/1 -> BK_CNT/1(Driver_Input), ENG_CNT/1(Driver_Input)
  BK_CNT/1(BK_CNT_out) -> Bus Creator1/4
  Bus Selector/5 -> BK_CNT/3(sensor_BK_PNT)  "<sensor_BK_PNT>"

== system TRAMI_STEP_AT_vehicle_ver01_Jmaab_R2018b_Intg/Vehicle/EL_PNT ==
  note: 低圧側電気負荷
  volt_BT_PNT_Lo_V : Inport
  Add : Sum  Inputs=+-
  Ground : Ground
  P_cal1 : METI_Lib_vehicle_model/P_cal  Type_energy=電気  Type_output_energy=損失  Power_name=Pl_  t_Workspace_Name=EL_PNT_ELEC_LOSS  P_VariableName=Pl_EL_PNT_ELEC_LOSS  Across_VariableName=V_EL_PNT_ELEC_LOSS  Throgh_VariableName=I_EL_PNT_ELEC_LOSS
  Product3 : Product  Inputs=*/  RndMeth=Zero
  Resistance2 : Constant  Value=EL_PNT_R_bodyelec_lo_ohm
  Terminator1 : Terminator
  current_EL_PNT_A : Outport
  wires:
  Product3/1 -> P_cal1/2, current_EL_PNT_A/1  "current_EL_PNT_A"
  volt_BT_PNT_Lo_V/1 -> Add/1
  Ground/1 -> Add/2
  Add/1 -> P_cal1/1, Product3/1
  Resistance2/1 -> Product3/2
  P_cal1/1 -> Terminator1/1

== system TRAMI_STEP_AT_vehicle_ver01_Jmaab_R2018b_Intg/Vehicle/ENG_PNT ==
  ENG_CNT_out : Inport
  w_ENG_PNT_radps : Inport  Port=2
  Bus Creator : BusCreator  Inputs=1
  Bus Selector7 : BusSelector  OutputSignals=open_throttle_per,flag_fuelcut,flag_IdleStop,timing_ignition
  ENG_Plant : Subsystem
  Memory : Memory
  sensor_ENG_PNT : Outport
  trq_ENG_PNT_Nm : Outport  Port=2
  wires:
  Memory/1 -> sensor_ENG_PNT/1  "sensor_ENG_PNT"
  w_ENG_PNT_radps/1 -> ENG_Plant/5(w_ENG_PNT_radps)
  ENG_Plant/2(trq_ENG_PNT_Nm) -> trq_ENG_PNT_Nm/1
  ENG_Plant/1(n_eng_rpm) -> Bus Creator/1
  ENG_CNT_out/1 -> Bus Selector7/1
  Bus Selector7/1 -> ENG_Plant/1(open_throttle_per)  "<open_throttle_per>"
  Bus Selector7/2 -> ENG_Plant/2(flag_fuelcut)  "<flag_fuelcut>"
  Bus Selector7/3 -> ENG_Plant/3(flag_IdleStop)  "<flag_IdleStop>"
  Bus Selector7/4 -> ENG_Plant/4(timing_ignition)  "<timing_ignition>"
  Bus Creator/1 -> Memory/1

== system TRAMI_STEP_AT_vehicle_ver01_Jmaab_R2018b_Intg/Vehicle/PTTH ==
  TM_CNT_out : Inport
  PHI_TM_PNT : Inport  Port=2
  v_VL_PNT_mps : Inport  Port=3
  ATM_PNT : Subsystem
  DTTH : Subsystem
  ENGTH : Subsystem
  RDTH_PNT : Subsystem
  T_TMTH_PNT : Outport
  wires:
  ENGTH/1(T_ENG_TM) -> DTTH/1(T_ENG_TM)
  RDTH_PNT/1(T_RD_TM) -> DTTH/5(T_RD_TM)
  ATM_PNT/1(T_ATM_TM) -> DTTH/6(T_ATM_TM)
  TM_CNT_out/1 -> DTTH/2(TM_CNT_out)
  PHI_TM_PNT/1 -> DTTH/3(PHI_TM_PNT)
  v_VL_PNT_mps/1 -> DTTH/4(v_VL_PNT_mps)
  DTTH/3(PHI_TM_RD) -> RDTH_PNT/1(PHI_TM_RD)
  DTTH/2(PHI_TM_ATM) -> ATM_PNT/1(PHI_TM_ATM)
  DTTH/4(PHI_TM_ENG) -> ENGTH/1(PHI_TM_ENG)
  DTTH/1(T_TMTH_PNT) -> T_TMTH_PNT/1

== system TRAMI_STEP_AT_vehicle_ver01_Jmaab_R2018b_Intg/Vehicle/ST_PNT ==
  ENG_CNT_out : Inport
  w_ENG_PNT_radps : Inport  Port=2
  volt_BT_PNT_Lo_V : Inport  Port=3
  Bus Selector1 : BusSelector  OutputSignals=flag_ON_Starter
  Constant1 : Constant  Value=OFF
  Constant6 : Constant  Value=OFF
  Gain : Gain  Gain=1/ST_PNT_Starter_Res_ohm
  Switch : Switch  Criteria=u2 > Threshold  Threshold=0.5
  Terminator : Terminator
  trq__ST_PNT_Nm : Outport
  current_ST_PNT_A : Outport  Port=2
  wires:
  volt_BT_PNT_Lo_V/1 -> Switch/1
  Switch/1 -> Gain/1
  Gain/1 -> current_ST_PNT_A/1  "current_ST_PNT_A"
  Constant6/1 -> Switch/3
  Constant1/1 -> trq__ST_PNT_Nm/1  "trq__ST_PNT_Nm"
  w_ENG_PNT_radps/1 -> Terminator/1
  ENG_CNT_out/1 -> Bus Selector1/1
  Bus Selector1/1 -> Switch/2  "<flag_ON_Starter>"

== system TRAMI_STEP_AT_vehicle_ver01_Jmaab_R2018b_Intg/Vehicle/TM_PNT ==
  TM_CNT_out : Inport
  trq_ENG_PNT_Nm : Inport  Port=2
  trq_ALT_PNT_Nm : Inport  Port=3
  trq__ST_PNT_Nm : Inport  Port=4
  w_TR_PNT_radps : Inport  Port=5
  T_TMTH_PNT : Inport  Port=6
  Memory : Memory
  Memory1 : Memory
  TM_PNT : Subsystem  TreatAsAtomicUnit=on
      settings: AttributesFormatString="<AtomicUnit =  %<TreatAsAtomicUnit>>"
  sensor_TM_PNT : Outport
  w_ENG_PNT_radps : Outport  Port=2
  trq_DS_PNT_Nm : Outport  Port=3
  PHI_TM_PNT : Outport  Port=4
  tag scope: TM_PNT_Info=global
  wires:
  Memory/1 -> sensor_TM_PNT/1  "sensor_TM_PNT"
  Memory1/1 -> w_ENG_PNT_radps/1  "w_ENG_PNT_radps"
  TM_CNT_out/1 -> TM_PNT/1(TM_CNT_out)
  trq_ENG_PNT_Nm/1 -> TM_PNT/2(trq_ENG_PNT_Nm)
  trq_ALT_PNT_Nm/1 -> TM_PNT/3(trq_ALT_PNT_Nm)
  trq__ST_PNT_Nm/1 -> TM_PNT/4(trq__ST_PNT_Nm)
  w_TR_PNT_radps/1 -> TM_PNT/5(w_TR_PNT_radps)
  T_TMTH_PNT/1 -> TM_PNT/6(T_TMTH_PNT)
  TM_PNT/5(TM_PNT_Info) -> [TM_PNT_Info]
  TM_PNT/4(PHI_TM_PNT) -> PHI_TM_PNT/1
  TM_PNT/2(trq_DS_PNT_Nm) -> trq_DS_PNT_Nm/1
  TM_PNT/3(w_ENG_PNT_radps) -> Memory1/1
  TM_PNT/1(sensor_TM_PNT) -> Memory/1

== system TRAMI_STEP_AT_vehicle_ver01_Jmaab_R2018b_Intg/Vehicle/TR_PNT ==
  note: 転がり抵抗
  note: 並進⇔回転変換
  note: トルク⇔力変換
  note: omg (回転数rad/s) = v (車速m/s) / r (タイヤ半径(m))
  note: M (トルクNm) = F (力(N)） × r (タイヤ半径(m))
  note: 車両を動かす側が正
  note: 車両を動かす側が正
  trq_DF_PNT_Nm : Inport
  trq_BK_PNT_Nm : Inport  Port=2
  v_VL_PNT_mps : Inport  Port=3
  Constant2 : Constant  Value=1/tire_r
  Product5 : Product  RndMeth=Zero
  Product6 : Product  RndMeth=Zero
  Q_cal1 : METI_Lib_vehicle_model/P_cal  Commented=on  Type_energy=並進運動  Type_output_energy=出力  Power_name=Po_  t_Workspace_Name=TR_PNT_MECK_DN  P_VariableName=Po_TR_PNT_MECK_DN  Across_VariableName=v_TR_PNT_MECK_DN  Throgh_VariableName=F_TR_PNT_MECK_DN
  Q_cal2 : METI_Lib_vehicle_model/P_cal  Commented=on  Type_energy=回転運動  Type_output_energy=出力  Power_name=Po_  t_Workspace_Name=TR_PNT_MECK_UP  P_VariableName=Po_TR_PNT_MECK_UP  Across_VariableName=w_TR_PNT_MECK_UP  Throgh_VariableName=tq_TR_PNT_MECK_UP
  Subtract2 : Sum
  Sum2 : Sum  Inputs=-+
  Terminator1 : Terminator  Commented=on
  Terminator2 : Terminator  Commented=on
  cal_roll_resi : METI_Lib_vehicle_model/vehicle_model/cal_roll_resi  Myu_tire=myu  Vehicle_Mass=M  Gravi_acc=g
  w_TR_PNT_radps : Outport
  f_TR_PNT_N : Outport  Port=2
  tag scope: tScope_Drive_Shaft_speed_rads=global
  wires:
  Sum2/1 -> f_TR_PNT_N/1  "f_TR_PNT_N"
  cal_roll_resi/1 -> Sum2/1, Q_cal1/2
  Product6/1 -> Sum2/2, Q_cal2/2
  Q_cal1/1 -> Terminator1/1
  Constant2/1 -> Product6/1, Product5/2
  v_VL_PNT_mps/1 -> Product5/1, cal_roll_resi/1, Q_cal1/1, Q_cal2/1
  Q_cal2/1 -> Terminator2/1
  Product5/1 -> [tScope_Drive_Shaft_speed_rads], w_TR_PNT_radps/1  "w_TR_PNT_radps"
  Subtract2/1 -> Product6/2  "trq_TR_in_Nm"
  trq_BK_PNT_Nm/1 -> Subtract2/2
  trq_DF_PNT_Nm/1 -> Subtract2/1

== system TRAMI_STEP_AT_vehicle_ver01_Jmaab_R2018b_Intg/Vehicle/VL_PNT ==
  note: 空気抵抗
  note: 車両慣性
  note: 登坂抵抗
  note: 車両を動かす側が正
  f_TR_PNT_N : Inport
  Bus Creator : BusCreator  Inputs=1
  Constant1 : Constant  Value=VL_PNT_Vehicle_Const
  Memory : Memory
  Product2 : Product
  Q_cal2 : METI_Lib_vehicle_model/P_cal  Type_energy=並進運動  Type_output_energy=出力  Power_name=Po_  t_Workspace_Name=VL_PNT_MASS_MECK  P_VariableName=Po_VL_PNT_MASS_MECK  Across_VariableName=v_VL_PNT_MASS_MECK  Throgh_VariableName=F_VL_PNT_MASS_MECK
  Q_cal3 : METI_Lib_vehicle_model/P_cal  Type_energy=並進運動  Type_output_energy=出力  Power_name=Po_  t_Workspace_Name=VL_PNT_MECK  P_VariableName=Po_VL_PNT_MECK  Across_VariableName=v_VL_PNT_MECK  Throgh_VariableName=F_VL_PNT_MECK
  Q_cal4 : METI_Lib_vehicle_model/P_cal  Type_energy=並進運動  Type_output_energy=損失  Power_name=Pl_  t_Workspace_Name=VL_PNT_Airresi_MECK_LOSS  P_VariableName=Pl_VL_PNT_Airresi_MECK_LOSS  Across_VariableName=v_VL_PNT_Airresi_MECK_LOSS  Throgh_VariableName=F_VL_PNT_Airresi_MECK_LOSS
  Sum1 : Sum  Inputs=-+
  Sum3 : Sum  Inputs=-+
  Terminator2 : Terminator
  Terminator3 : Terminator
  Terminator4 : Terminator  Commented=on
  To Workspace3 : ToWorkspace  VariableName=Q_GradrResi  SaveFormat=Structure With Time  SampleTime=-1
      settings: Decimation=100
  V_wind : Constant  Value=VL_PNT_V_wind
  cal_Air_resi : METI_Lib_vehicle_model/vehicle_model/cal_Air_resi  Vel_max=vel_max
  cal_Vehicle_Mass : METI_Lib_vehicle_model/vehicle_model/cal_Vehicle_Mass  Vehicle_Mass=M
  mps2kmph : Gain  Gain=mps2kmph
  sensor_VL_PNT : Outport
  v_VL_PNT_mps : Outport  Port=2
  wires:
  Product2/1 -> To Workspace3/1
  Sum3/1 -> Sum1/2
  Sum1/1 -> Q_cal2/2, cal_Vehicle_Mass/1
  cal_Vehicle_Mass/1 -> v_VL_PNT_mps/1, Q_cal3/1, cal_Air_resi/1, Q_cal4/1, Product2/1, mps2kmph/1, Q_cal2/1  "v_VL_PNT_mps"
  cal_Air_resi/1 -> Q_cal4/2, Sum3/1
  V_wind/1 -> cal_Air_resi/2
  Constant1/1 -> Sum1/1, Product2/2
  Q_cal2/1 -> Terminator2/1
  Q_cal3/1 -> Terminator3/1
  Q_cal4/1 -> Terminator4/1
  mps2kmph/1 -> Bus Creator/1  "v_VL_PNT_kmph"
  f_TR_PNT_N/1 -> Sum3/2, Q_cal3/2
  Bus Creator/1 -> Memory/1
  Memory/1 -> sensor_VL_PNT/1  "sensor_VL_PNT"

== system TRAMI_STEP_AT_vehicle_ver01_Jmaab_R2018b_Intg/Driver/Caliculate_Opeining_Accel/FB ==
  delta_v_VL_kmph : Inport
  Acc_D_Gain : Gain  Gain=D_Gain
  Acc_I_Gain : Gain  Gain=I_Gain
  Acc_P_Gain : Gain  Gain=P_Gain
  Acc_P_Gain1 : Gain  Gain=P_Gain
  Derivative : Derivative
  Filter : Subsystem  Commented=through
  Integrator : Integrator
  Memory : Memory
  Product1 : Product
  Saturation2 : Saturate  UpperLimit=1  LowerLimit=0
  Sum : Sum  Inputs=+++
  Terminator : Terminator
  FB_open_accel_per : Outport
  wires:
  Filter/1(Out1) -> Product1/2
  Saturation2/1 -> Acc_P_Gain/1
  Acc_P_Gain/1 -> Product1/1
  Sum/1 -> FB_open_accel_per/1
  Derivative/1 -> Acc_D_Gain/1
  Integrator/1 -> Acc_I_Gain/1
  delta_v_VL_kmph/1 -> Memory/1
  Acc_I_Gain/1 -> Sum/3
  Acc_D_Gain/1 -> Sum/2
  Product1/1 -> Sum/1
  Memory/1 -> Saturation2/1, Filter/1(In1), Acc_P_Gain1/1, Integrator/1, Derivative/1
  Acc_P_Gain1/1 -> Terminator/1

== system TRAMI_STEP_AT_vehicle_ver01_Jmaab_R2018b_Intg/Driver/Caliculate_Opeining_Accel/FF ==
  note: 速度とパワーでF/B出来るようにモデルを用意しておく
      | 切り替えスイッチを作っておく
  v_VL_PNT_kmph : Inport
  target_v_VL_kmph : Inport  Port=2
  pre_n_eng_rpm : Inport  Port=3
  pre_ratio_DCT : Inport  Port=4
  Air_Resistance : Subsystem
  Cal_M_ENG_jiku2 : Subsystem
  Constant : Constant  Value=0.1
  Constant3 : Constant  Value=tire_r
  Constant4 : Constant  Value=TM_PNT_FD_gear
  Inertial_Resistance : Subsystem
  MinMax : MinMax  Function=max  Inputs=2
  Product8 : Product  Inputs=*/*/  RndMeth=Zero
  Rolling_Resistance : Subsystem
  Sum4 : Sum  Inputs=+++
  Terminator : Terminator
  kmph2mps : Gain  Gain=kmph2mps
  kmph2mps1 : Gain  Gain=kmph2mps
  FF_open_accel_per : Outport
  wires:
  kmph2mps/1 -> Inertial_Resistance/1(V_tgt), Rolling_Resistance/1(V_tgt), Air_Resistance/1(V_tgt)
  target_v_VL_kmph/1 -> kmph2mps/1
  Sum4/1 -> Product8/1
  Constant4/1 -> Product8/2
  Constant3/1 -> Product8/3
  Air_Resistance/1(F_air_resi) -> Sum4/2
  Rolling_Resistance/1(F_rollresi) -> Sum4/3
  Inertial_Resistance/1(F_Inertia) -> Sum4/1
  pre_ratio_DCT/1 -> MinMax/2
  v_VL_PNT_kmph/1 -> kmph2mps1/1
  kmph2mps1/1 -> Terminator/1
  Cal_M_ENG_jiku2/1(FF_open_accel_per) -> FF_open_accel_per/1
  Product8/1 -> Cal_M_ENG_jiku2/1(FF_trq_accel_Nm)  "FF_trq_accel_Nm"
  pre_n_eng_rpm/1 -> Cal_M_ENG_jiku2/2(pre_n_eng_rpm)
  Constant/1 -> MinMax/1
  MinMax/1 -> Product8/4

== system TRAMI_STEP_AT_vehicle_ver01_Jmaab_R2018b_Intg/Vehicle/ALT_PNT/Subsystem ==
  note: V_ALT_PNT
  note: オルタ要求トルク上限/下限ガード処理追加
      | (低回転数、低電流時に要求トルクが過大となるのを防止するため
      |  :マップの外挿方法が線形となっていることが原因)
  target_volt_ALT_V : Inport
  w_ROT_slavepulley12 : Inport  Port=2
  volt_BT_PNT_Lo_V : Inport  Port=3
  Constant1 : Constant  Value=ALT_PNT_ALT_GDCurrent_A
  Constant2 : Constant  Value=ALT_PNT_ALT_GDVolt_V
  I_alt_cal : Subsystem
  Torque_Guard : Subsystem
  Transfer Fcn1 : TransferFcn  Denominator=|
      | [ALT_PNT_Tau_Alternator_trq_Nm
      |  1]
  omg2rpm : Gain  Gain=radpsec2rpm
  current_ALT_PNT_A : Outport
  trq_trqsource : Outport  Port=2
  wires:
  I_alt_cal/1(I_alt) -> Torque_Guard/1(current_ALT_PNT_A), current_ALT_PNT_A/1  "current_ALT_PNT_A"
  target_volt_ALT_V/1 -> I_alt_cal/1(target_volt_ALT_V)
  volt_BT_PNT_Lo_V/1 -> Torque_Guard/2(V_ALT_PNT), I_alt_cal/2(volt_BT_PNT_Lo_V)
  Transfer Fcn1/1 -> trq_trqsource/1
  omg2rpm/1 -> Torque_Guard/3(n_ROT_slavepulley12_rpm), I_alt_cal/3(rpm_alt)  "n_ROT_slavepulley12_rpm"
  w_ROT_slavepulley12/1 -> omg2rpm/1
  Constant1/1 -> Torque_Guard/4(ALT_GDCurrent)
  Constant2/1 -> Torque_Guard/5(ALT_GDVolt)
  Torque_Guard/1(trq_trqsource) -> Transfer Fcn1/1

== system TRAMI_STEP_AT_vehicle_ver01_Jmaab_R2018b_Intg/Vehicle/ALT_PNT/pulley_slave ==
  note: プーリー比
  note: プーリー効率
  w_ENG_PNT_radps : Inport
  trq_slavepulley12 : Inport  Port=2
  Goto3 : Goto  Commented=on  GotoTag=tScope_pulley1Loss  TagVisibility=global
  P_cal : AZAPA_Lib_vehicle_model/P_cal  Commented=on  Type_energy=並進運動  Type_output_energy=出力  Power_name=Po_  t_Workspace_Name=MOTOR_MECK  P_VariableName=Po_MOTOR_MECK  Across_VariableName=v_MOTOR_MECK  Throgh_VariableName=F_MOTOR_MECK
  Product : Product  RndMeth=Zero
  Product1 : Product  RndMeth=Zero
  eta_cal2 : METI_Lib_vehicle_model/eta_cal2  SystemSampleTime=-1
  eta_pulley : Constant  Value=ALT_PNT_eta_pulley_alt
  ratio_pulley : Constant  Value=ALT_PNT_ratio_pulley_alt
  trq_slavepulley11 : Outport
  w_slavepulley12 : Outport  Port=2
  wires:
  eta_cal2/1 -> P_cal/2
  P_cal/1 -> Goto3/1
  w_ENG_PNT_radps/1 -> P_cal/1, Product1/1
  eta_cal2/2 -> trq_slavepulley11/1
  trq_slavepulley12/1 -> Product/2
  eta_pulley/1 -> eta_cal2/1
  Product1/1 -> w_slavepulley12/1
  ratio_pulley/1 -> Product/1, Product1/2
  Product/1 -> eta_cal2/2

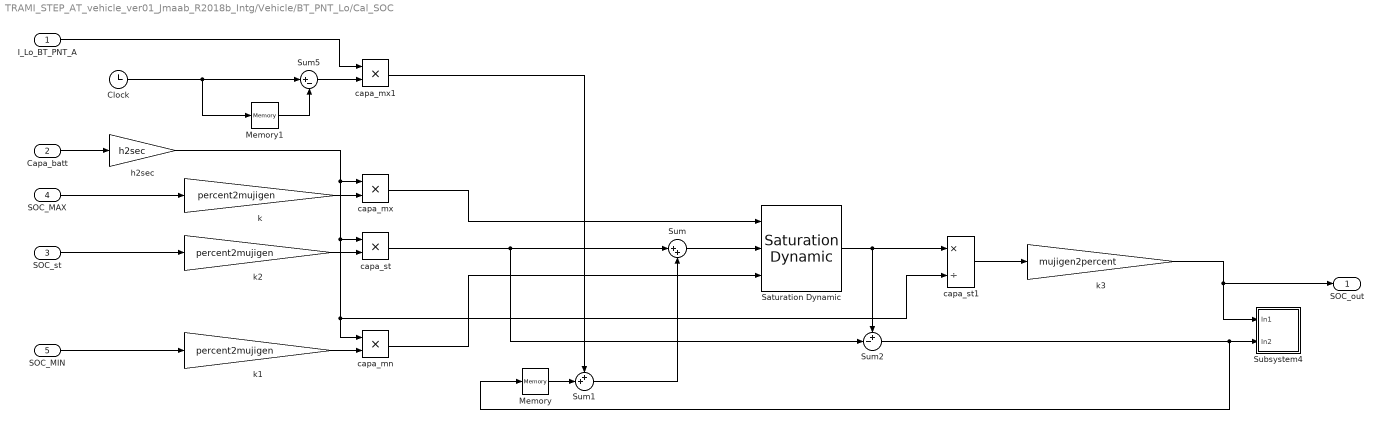
== system TRAMI_STEP_AT_vehicle_ver01_Jmaab_R2018b_Intg/Vehicle/BT_PNT_Lo/Cal_SOC ==
  I_Lo_BT_PNT_A : Inport
  Capa_batt : Inport  Port=2
  SOC_st : Inport  Port=3
  SOC_MAX : Inport  Port=4
  SOC_MIN : Inport  Port=5
  Clock : Clock
  Memory : Memory
  Memory1 : Memory
  Saturation Dynamic : simulink/Discontinuities/Saturation Dynamic  OutMin=[]  OutMax=[]  OutDataTypeStr=Inherit: Same as second input  OutDataType=fixdt(1, 16)  OutScaling=2^-10  DoSatur=off
  Subsystem4 : Subsystem  mask{SOC=SOC_LoBat, VariableName=Asec_LoBat}
      mask prompts: SOC "バッテリSOC"; VariableName "バッテリ容量変化量(Asec)"
  Sum : Sum  Inputs=|++
  Sum1 : Sum  Inputs=++|
  Sum2 : Sum  Inputs=+-|
  Sum5 : Sum  Inputs=|+-
  capa_mn : Product  RndMeth=Zero
  capa_mx : Product  RndMeth=Zero
  capa_mx1 : Product  RndMeth=Zero
  capa_st : Product  RndMeth=Zero
  capa_st1 : Product  Inputs=*/  RndMeth=Zero
  h2sec : Gain  Gain=h2sec
  k : Gain  Gain=percent2mujigen
  k1 : Gain  Gain=percent2mujigen
  k2 : Gain  Gain=percent2mujigen
  k3 : Gain  Gain=mujigen2percent
  SOC_out : Outport
  wires:
  Sum5/1 -> capa_mx1/2
  Memory1/1 -> Sum5/2
  Sum/1 -> Saturation Dynamic/2
  Clock/1 -> Sum5/1, Memory1/1
  capa_mx1/1 -> Sum1/1
  k3/1 -> Subsystem4/1(In1), SOC_out/1
  Sum1/1 -> Sum/2
  Memory/1 -> Sum1/2
  k2/1 -> capa_st/2
  k1/1 -> capa_mn/2
  k/1 -> capa_mx/2
  capa_st/1 -> Sum2/2, Sum/1
  Saturation Dynamic/1 -> Sum2/1, capa_st1/1
  capa_mx/1 -> Saturation Dynamic/1
  capa_mn/1 -> Saturation Dynamic/3
  capa_st1/1 -> k3/1
  h2sec/1 -> capa_mn/1, capa_st1/2, capa_st/1, capa_mx/1
  SOC_MIN/1 -> k1/1
  SOC_MAX/1 -> k/1
  SOC_st/1 -> k2/1
  Capa_batt/1 -> h2sec/1
  I_Lo_BT_PNT_A/1 -> capa_mx1/1
  Sum2/1 -> Memory/1, Subsystem4/2(In2)

== system TRAMI_STEP_AT_vehicle_ver01_Jmaab_R2018b_Intg/Vehicle/BT_PNT_Lo/Subsystem ==
  I_BT_PNT_Lo_A : Inport
  Divide : Product
  Resistivity : Constant  Value=BT_PNT_Lo_R_lo_batt_ohm
  Sum : Sum  Inputs=|++
  Transfer Fcn : TransferFcn  Numerator=[0.01]  Denominator=[0.1 1]
  V_BT_PNT_Lo_V : Outport
  wires:
  Resistivity/1 -> Divide/2
  Divide/1 -> Sum/1
  I_BT_PNT_Lo_A/1 -> Divide/1, Transfer Fcn/1
  Sum/1 -> V_BT_PNT_Lo_V/1
  Transfer Fcn/1 -> Sum/2

== system TRAMI_STEP_AT_vehicle_ver01_Jmaab_R2018b_Intg/Vehicle/CNT/ALT_CNT ==
  sensor_BT_PNT_Lo_BUS : Inport
  ALT_Ctrl : Subsystem
  Bus Creator6 : BusCreator  Inputs=1
  Bus Selector1 : BusSelector  OutputSignals=flag_fuelcut,flag_IdleStop,n_eng_rpm
  Bus Selector9 : BusSelector  OutputSignals=SOC_BT_PNT_Lo_PCT
  ALT_CNT_out : Outport
  wires:
  [ALT_CNT_CAN_Rx] -> Bus Selector1/1
  Bus Selector1/1 -> ALT_Ctrl/2(flag_fuelcut)  "<flag_fuelcut>"
  Bus Selector1/2 -> ALT_Ctrl/3(flag_IdleStop)  "<flag_IdleStop>"
  Bus Selector1/3 -> ALT_Ctrl/4(n_eng_rpm)  "<n_eng_rpm>"
  ALT_Ctrl/1(target_volt_ALT_V) -> Bus Creator6/1
  sensor_BT_PNT_Lo_BUS/1 -> Bus Selector9/1
  Bus Selector9/1 -> ALT_Ctrl/1(SOC_BT_PNT_Lo_PCT)  "<SOC_BT_PNT_Lo_PCT>"
  Bus Creator6/1 -> ALT_CNT_out/1  "ALT_CNT_out"

== system TRAMI_STEP_AT_vehicle_ver01_Jmaab_R2018b_Intg/Vehicle/CNT/BK_CNT ==
  Driver_Input : Inport
  sensor_VL_PNT : Inport  Port=2
  sensor_BK_PNT : Inport  Port=3
  BK_Ctrl : Subsystem
  Bus Creator1 : BusCreator  Inputs=1
  Bus Creator2 : BusCreator  Inputs=2
  Bus Selector1 : BusSelector  OutputSignals=trq_BK_PNT_Nm
  Bus Selector12 : BusSelector  OutputSignals=v_VL_PNT_kmph
  Bus Selector4 : BusSelector  OutputSignals=open_brake_per
  BK_CNT_out : Outport
  tag scope: BK_CNT_CAN_Tx=scoped
  wires:
  BK_Ctrl/1(open_brake_per) -> Bus Creator1/1
  Driver_Input/1 -> Bus Selector4/1
  Bus Selector4/1 -> BK_Ctrl/1(open_brake_per_in)  "<open_brake_per>"
  Bus Creator1/1 -> BK_CNT_out/1  "BK_CNT_out"
  sensor_BK_PNT/1 -> Bus Selector1/1
  Bus Selector1/1 -> BK_Ctrl/3(trq_BK_PNT_Nm_in)  "<trq_BK_PNT_Nm>"
  Bus Creator2/1 -> [BK_CNT_CAN_Tx]  "BK_CNT_CAN_Tx"
  BK_Ctrl/3(trq_BK_PNT_Nm) -> Bus Creator2/2
  sensor_VL_PNT/1 -> Bus Selector12/1
  Bus Selector12/1 -> BK_Ctrl/2(v_VL_PNT_kmph_in)  "<v_VL_PNT_kmph>"
  BK_Ctrl/2(v_VL_PNT_kmph) -> Bus Creator2/1

== system TRAMI_STEP_AT_vehicle_ver01_Jmaab_R2018b_Intg/Vehicle/CNT/CAN ==
  note: CAN Bus Model
  ALT_CNT : Subsystem
  BK_CNT : Subsystem
  ENG_CNT : Subsystem
  Pwtr_CAN : Subsystem
  TM_CNT : Subsystem
  wires:
  Pwtr_CAN/1(Pwtr_CAN) -> BK_CNT/1(Pwtr_CAN), ALT_CNT/1(Pwtr_CAN), ENG_CNT/1(Pwtr_CAN), TM_CNT/1(Pwtr_CAN)
  ENG_CNT/1(ENG_CNT_CAN_Tx) -> Pwtr_CAN/1(ENG_CNT_CAN_Tx)
  TM_CNT/1(TM_CNT_CAN_Tx) -> Pwtr_CAN/2(TM_CNT_CAN_Tx)
  BK_CNT/1(BK_CNT_CAN_Tx) -> Pwtr_CAN/3(BK_CNT_CAN_Tx)

== system TRAMI_STEP_AT_vehicle_ver01_Jmaab_R2018b_Intg/Vehicle/CNT/ENG_CNT ==
  Driver_Input : Inport
  sensor_ENG_PNT : Inport  Port=2
  Bus Creator : BusCreator  Inputs=6
  Bus Creator1 : BusCreator  Inputs=7
  Bus Selector1 : BusSelector  OutputSignals=v_VL_PNT_kmph,flag_lock_up
  Bus Selector13 : BusSelector  OutputSignals=n_eng_rpm
  Bus Selector14 : BusSelector  OutputSignals=open_accel_per,open_brake_per
  ENG_Cntrl : Subsystem
  ENG_CNT_out : Outport
  tag scope: ENG_CNT_CAN_Tx=scoped
  wires:
  Bus Creator/1 -> [ENG_CNT_CAN_Tx]  "ENG_CNT_CAN_Tx"
  Bus Selector1/2 -> ENG_Cntrl/5(flag_Lockup)  "<flag_lock_up>"
  ENG_Cntrl/1(open_throttle_per) -> Bus Creator/1, Bus Creator1/1
  ENG_Cntrl/2(flag_IdleStop) -> Bus Creator/2, Bus Creator1/2
  ENG_Cntrl/3(flag_fuelcut) -> Bus Creator/3, Bus Creator1/3
  ENG_Cntrl/4(fuel_ratio) -> Bus Creator1/4
  ENG_Cntrl/5(timing_ignition) -> Bus Creator1/5
  ENG_Cntrl/6(n_eng_rpm) -> Bus Creator/4, Bus Creator1/6
  ENG_Cntrl/7(flag_ON_Starter) -> Bus Creator1/7
  Bus Creator1/1 -> ENG_CNT_out/1  "ENG_CNT_out"
  sensor_ENG_PNT/1 -> Bus Selector13/1
  Bus Selector13/1 -> ENG_Cntrl/1(sens_ENG_PNT)  "<n_eng_rpm>"
  Driver_Input/1 -> Bus Selector14/1
  Bus Selector14/1 -> Bus Creator/6, ENG_Cntrl/3(open_accel_per)  "<open_accel_per>"
  Bus Selector14/2 -> ENG_Cntrl/4(open_brake_per)  "<open_brake_per>"
  [ENG_CNT_CAN_Rx] -> Bus Selector1/1
  ENG_Cntrl/8(IdleSpeed_Target) -> Bus Creator/5
  Bus Selector1/1 -> ENG_Cntrl/2(v_VL_PNT_kmph)  "<v_VL_PNT_kmph>"

== system TRAMI_STEP_AT_vehicle_ver01_Jmaab_R2018b_Intg/Vehicle/CNT/TM_CNT ==
  sensor_TM_PNT_BUS : Inport
  Rate Transition : RateTransition  Deterministic=off
      settings: AttributesFormatString=|
      | <Integrity = %<Integrity>>
      | <Deterministic = %<Deterministic>>
  Rate Transition1 : RateTransition  Deterministic=off
      settings: AttributesFormatString=|
      | <Integrity = %<Integrity>>
      | <Deterministic = %<Deterministic>>
  Rate Transition2 : RateTransition  Deterministic=off
      settings: AttributesFormatString=|
      | <Integrity = %<Integrity>>
      | <Deterministic = %<Deterministic>>
  TM_CNT : Subsystem  TreatAsAtomicUnit=on
      settings: AttributesFormatString="<AtomicUnit =  %<TreatAsAtomicUnit>>"
  TM_CNT_out : Outport
  tag scope: TM_CNT_CAN_Tx=scoped, TM_CNT_Info=global
  wires:
  sensor_TM_PNT_BUS/1 -> Rate Transition/1
  [TM_CNT_CAN_Rx] -> Rate Transition1/1
  TM_CNT/1(TM_CNT_out) -> Rate Transition2/1
  TM_CNT/2(TM_CNT_CAN_Tx) -> [TM_CNT_CAN_Tx]
  TM_CNT/3(TM_CNT_Info) -> [TM_CNT_Info]
  Rate Transition/1 -> TM_CNT/1(sensor_TM_PNT_BUS)
  Rate Transition1/1 -> TM_CNT/2(TM_CNT_CAN_Rx)
  Rate Transition2/1 -> TM_CNT_out/1  "TM_CNT_out"
